simulink model "simple_MAV_alternative_Simulink"  (R2019a)
settings: Solver=ode4  StartTime=0.0  StopTime=50  FixedStep=P.Ts  RelTol=1e-3
settings Model: Creator=simao  LastModifiedBy=Hugo Pereira

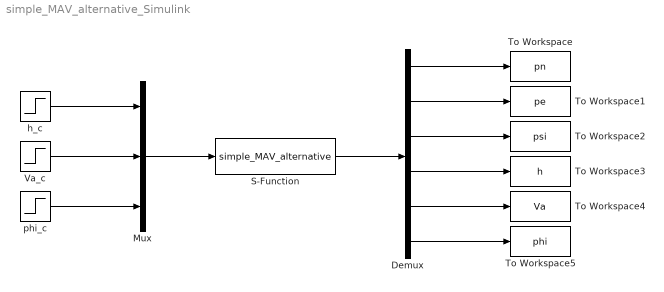
== system simple_MAV_alternative_Simulink ==
  Demux : Demux  Outputs=6
  Mux : Mux  Inputs=3
  S-Function : S-Function  FunctionName=simple_MAV_alternative  Parameters=P  SFunctionDeploymentMode=off  EnableBusSupport=off
  To Workspace : ToWorkspace  VariableName=pn  SaveFormat=Timeseries  SampleTime=-1
  To Workspace1 : ToWorkspace  VariableName=pe  SaveFormat=Timeseries  SampleTime=-1
  To Workspace2 : ToWorkspace  VariableName=psi  SaveFormat=Timeseries  SampleTime=-1
  To Workspace3 : ToWorkspace  VariableName=h  SaveFormat=Timeseries  SampleTime=-1
  To Workspace4 : ToWorkspace  VariableName=Va  SaveFormat=Timeseries  SampleTime=-1
  To Workspace5 : ToWorkspace  VariableName=phi  SaveFormat=Timeseries  SampleTime=-1
  Va_c : Step  Time=0  After=20  SampleTime=0
  h_c : Step  Time=0  After=100  SampleTime=0
  phi_c : Step  Time=0  After=5*pi/180  SampleTime=0
  wires:
  Mux/1 -> S-Function/1
  Demux/5 -> To Workspace4/1
  Demux/4 -> To Workspace3/1
  Demux/3 -> To Workspace2/1
  S-Function/1 -> Demux/1
  Demux/1 -> To Workspace/1
  Demux/2 -> To Workspace1/1
  Demux/6 -> To Workspace5/1
  h_c/1 -> Mux/1
  Va_c/1 -> Mux/2
  phi_c/1 -> Mux/3
